simulink model "run_first"  (R2024b)
settings: Solver=ode1  StartTime=0.0  StopTime=70  FixedStep=0.001  RelTol=1e-3
values from neighbouring files (symbols this model uses):
  b = 0.000178    [Controller.m]    (also in FeetForward_Controller.mat; ReactionWheelModel1.m; run_FIRST.m = 3.97e-06)
  g = 9.81    [run_FIRST.m]
  GR = 2.5    [run_FIRST.m]
  i_0 = 0    [run_FIRST.m]
  J = 0.00725    [Controller.m]    (also in FeetForward_Controller.mat; ReactionWheelModel1.m; run_FIRST.m = 0.0001)
  Kb = 0.01    [Model_2811.m]    (also in run_FIRST.m = 0.00574)
  Km = 0.01    [Model_2811.m]    (also in run_FIRST.m = 0.00574)
  L = 0.00339    [Controller.m]    (also in FeetForward_Controller.mat; Model_2811.m = 0.001; ReactionWheelModel1.m; run_FIRST.m = 0.003)
  m = 1.136    [run_FIRST.m]
  Q = 0.37    [run_FIRST.m]
  R = 1.52    [Controller.m]    (also in FeetForward_Controller.mat; Model_2811.m = 1; ReactionWheelModel1.m; run_FIRST.m = 0.141)
  Rw = 3.2e-2    (= 0.032)    [run_FIRST.m]
  tht_0 = 0    [run_FIRST.m]
  tol = 1.0e-10    (= 1e-10)    [run_FIRST.m]
  v_0 = 0    [run_FIRST.m]
  wm_0 = 0    [run_FIRST.m]
  wm_des = 275    [run_FIRST.m]
  xp_0 = 0    [run_FIRST.m]
libraries: simulink x1
settings Model: Creator=LEGION  LastModifiedBy=LEGION

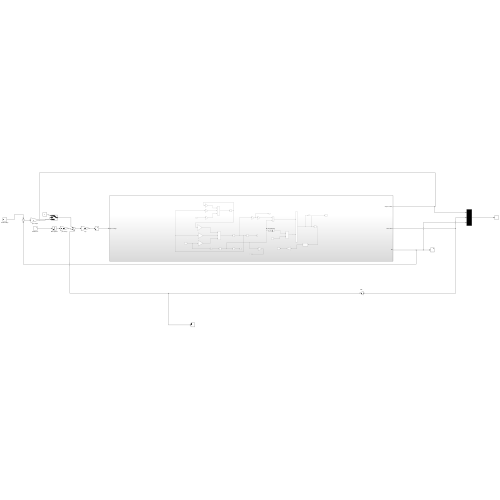
[thumbnail: Simulink's stored preview of the top-level diagram]
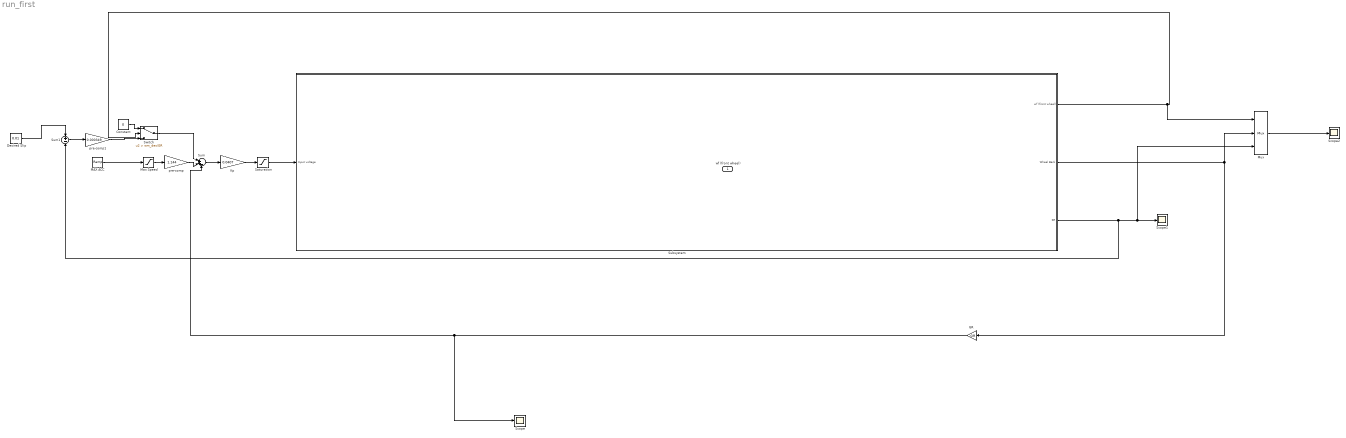
== system run_first ==
  Constant : Constant  Value=0
  Desired Slip : Constant  Value=0.01
  GR : Gain  Gain=GR
  Kp : Gain  Gain=0.0407
  MAX ACC : simulink/Sources/Ramp  slope=50  start=0  InitialOutput=0
  Max Speed : Saturate  UpperLimit=wm_des
  Mux : Mux  Inputs=3
  Saturation : Saturate  UpperLimit=12  LowerLimit=0
  Scope : Scope
  Scope1 : Scope
  Scope2 : Scope
  Subsystem : Subsystem
  Sum : Sum  Inputs=|++-
  Sum1 : Sum  Inputs=+-
  Switch : Switch  Criteria=u2 > Threshold  Threshold=wm_des/GR  SaturateOnIntegerOverflow=off  InputSameDT=off
  pre-comp : Gain  Gain=1.144
  pre-comp1 : Gain  Gain=0.000349
  wf (front wheel) : Outport
  wires:
  Subsystem/2(Wheel Back) -> Mux/2, GR/1
  GR/1 -> Sum/3, Scope/1
  MAX ACC/1 -> Max Speed/1
  Saturation/1 -> Subsystem/1(Input voltage)
  Max Speed/1 -> pre-comp/1
  pre-comp/1 -> Sum/2
  Kp/1 -> Saturation/1
  Sum/1 -> Kp/1
  Switch/1 -> Sum/1
  Subsystem/1(wf (front wheel)) -> Mux/1, Switch/2
  Constant/1 -> Switch/1
  Sum1/1 -> pre-comp1/1
  Desired Slip/1 -> Sum1/1
  Subsystem/3(SR) -> Mux/3, Scope1/1, Sum1/2
  pre-comp1/1 -> Switch/3
  Mux/1 -> Scope2/1

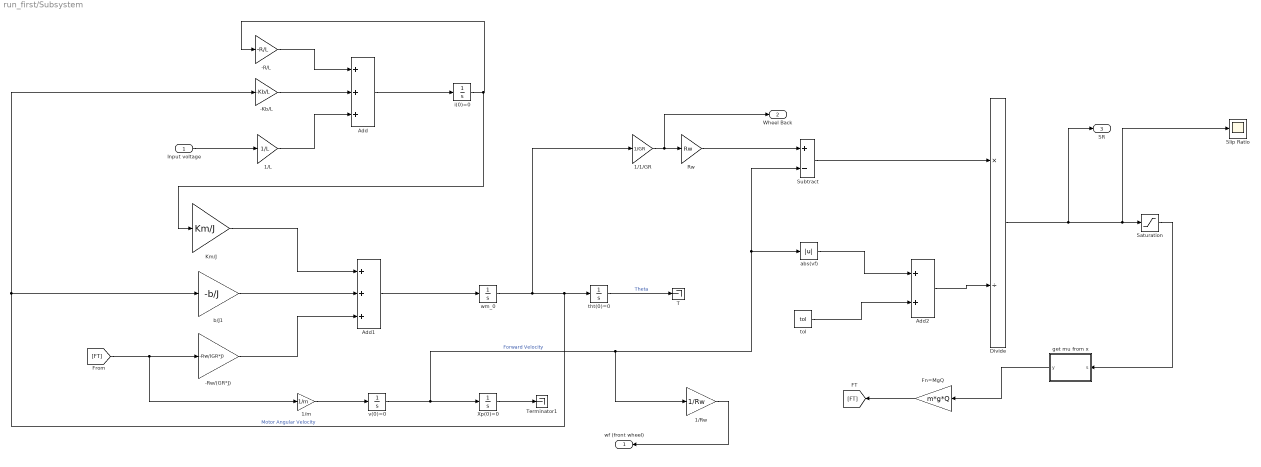
== system run_first/Subsystem ==
  Input voltage : Inport
  -Kb/L : Gain  Gain=-Kb/L
  -R/L : Gain  Gain=-R/L
  -Rw/(GR*J) : Gain  Gain=-Rw/(GR*J)
  1/1/GR : Gain  Gain=1/GR
  1/L : Gain  Gain=1/L
  1/Rw : Gain  Gain=1/Rw
  1/m : Gain  Gain=1/m
  Add : Sum  Inputs=+++
  Add1 : Sum  Inputs=+++
  Add2 : Sum
  Divide : Product  Inputs=*/
  Fn=MgQ : Gain  Gain=m*g*Q
  Km/J : Gain  Gain=Km/J
  Rw : Gain  Gain=Rw
  Saturation : Saturate  UpperLimit=1  LowerLimit=-1
  Slip Ratio : Scope
  Subtract : Sum  Inputs=+-
  T : Terminator
  Terminator1 : Terminator
  Xp(0)=0 : Integrator  InitialCondition=xp_0
  abs(vf) : Abs  SaturateOnIntegerOverflow=off
  b/J1 : Gain  Gain=-b/J
  get mu from x : MATLAB Function  TreatAsAtomicUnit=on
  i(0)=0 : Integrator  InitialCondition=i_0
  tht(0)=0 : Integrator  InitialCondition=tht_0
  tol : Constant  Value=tol
  v(0)=0 : Integrator  InitialCondition=v_0
  wm_0 : Integrator  InitialCondition=wm_0
  wf (front wheel) : Outport
  Wheel Back : Outport  Port=2
  SR : Outport  Port=3
  wires:
  Input voltage/1 -> 1/L/1
  1/L/1 -> Add/3
  Subtract/1 -> Divide/1
  wm_0/1 -> 1/1/GR/1, -Kb/L/1, b/J1/1, tht(0)=0/1  "Motor Angular Velocity"
  abs(vf)/1 -> Add2/1
  Add2/1 -> Divide/2
  tol/1 -> Add2/2
  Rw/1 -> Subtract/1
  1/1/GR/1 -> Wheel Back/1, Rw/1
  i(0)=0/1 -> Km/J/1, -R/L/1
  Fn=MgQ/1 -> [FT]
  1/Rw/1 -> wf (front wheel)/1
  v(0)=0/1 -> 1/Rw/1, abs(vf)/1, Subtract/2, Xp(0)=0/1  "Forward Velocity"
  Xp(0)=0/1 -> Terminator1/1
  Add1/1 -> wm_0/1
  Add/1 -> i(0)=0/1
  Saturation/1 -> get mu from x/1(s)
  -R/L/1 -> Add/1
  1/m/1 -> v(0)=0/1
  [FT] -> 1/m/1, -Rw/(GR*J)/1
  b/J1/1 -> Add1/2
  Km/J/1 -> Add1/1
  -Rw/(GR*J)/1 -> Add1/3
  tht(0)=0/1 -> T/1  "Theta"
  get mu from x/1(y) -> Fn=MgQ/1
  Divide/1 -> SR/1, Slip Ratio/1, Saturation/1
  -Kb/L/1 -> Add/2

== matlab function run_first/Subsystem/get mu from x ==
  data: y output; s input
function y = fcn(s)
%#codegen

%slip is already saturated
%ONLY DEFINED from 1 to -1

a1=1.63;
a2=-0.9;
a3=-0.1;

c1=-27;
c2=-15;

if s<0
    s=abs(s);
    mu=-(a1*(1-exp(c1*s))+a2*(1-exp(c2*s))+a3*s);
else
    mu=a1*(1-exp(c1*s))+a2*(1-exp(c2*s))+a3*s;
end

y = mu;
